simulink model "passive_cellBalancing"  (R2021a)
settings: Solver=VariableStepAuto  StartTime=0.0  StopTime=4000  RelTol=1e-3
undefined symbols (not defined in the file or in its folder): Ion, Lithium
libraries: spsBatteryLib x4, spsMosfetLib x4, spsSeriesRLCBranchLib x4, spspowerguiLib x1
settings Model: EnablePacing=on  PacingRate=100  Creator=Navadeep  LastModifiedBy=Navadeep

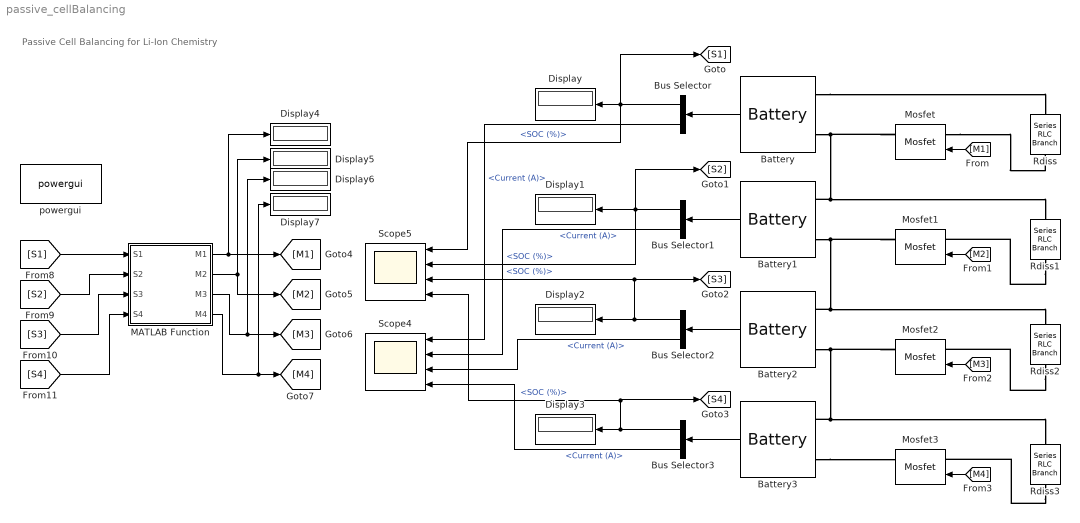
== system passive_cellBalancing ==
  note: Passive Cell Balancing for Li-Ion Chemistry
  Battery : spsBatteryLib/Battery  BatType=Lithium-Ion  ShowTempParam=off  ThermalPreset=no  ShowAgeParam=off  NomV=3.7  NomQ=7.5  SOC=70  Batt_Tr=30  PresetModel=on  MaxQ=7.5  MinV=2.775  FullV=4.3068  Dis_rate=3.2609  R=0.0049333  Normal_OP=6.7826  expZone="[3.9974     0.36848]"  current=[6.5 13 32.5]  Units=Time  Tci=20  NomT=20  T2=-30  MaxQ2=4.8  FullV2=7.1  Normal_OP2=5.655  expZone2="[6.58           1]"  Rca=0.6  ti=2000  Dp=0  Neq0=0  Tsim=1e6  Ta1=25  Qeol=5.4*0.9  Reol=0.013333*1.2  Char_age=[2.3478, 3]  Dis_age=[2.3478, 10]  N1=1500  N2=10500  N3=1000  N4=1400  Ta2=45  N5=950
  Battery1 : spsBatteryLib/Battery  BatType=Lithium-Ion  ShowTempParam=off  ThermalPreset=no  ShowAgeParam=off  NomV=3.7  NomQ=7.5  SOC=80  Batt_Tr=30  PresetModel=on  MaxQ=7.5  MinV=2.775  FullV=4.3068  Dis_rate=3.2609  R=0.0049333  Normal_OP=6.7826  expZone="[3.9974     0.36848]"  current=[6.5 13 32.5]  Units=Time  Tci=20  NomT=20  T2=-30  MaxQ2=4.8  FullV2=7.1  Normal_OP2=5.655  expZone2="[6.58           1]"  Rca=0.6  ti=2000  Dp=0  Neq0=0  Tsim=1e6  Ta1=25  Qeol=5.4*0.9  Reol=0.013333*1.2  Char_age=[2.3478, 3]  Dis_age=[2.3478, 10]  N1=1500  N2=10500  N3=1000  N4=1400  Ta2=45  N5=950
  Battery2 : spsBatteryLib/Battery  BatType=Lithium-Ion  ShowTempParam=off  ThermalPreset=no  ShowAgeParam=off  NomV=3.7  NomQ=7.5  SOC=75  Batt_Tr=30  PresetModel=on  MaxQ=7.5  MinV=2.775  FullV=4.3068  Dis_rate=3.2609  R=0.0049333  Normal_OP=6.7826  expZone="[3.9974     0.36848]"  current=[6.5 13 32.5]  Units=Time  Tci=20  NomT=20  T2=-30  MaxQ2=4.8  FullV2=7.1  Normal_OP2=5.655  expZone2="[6.58           1]"  Rca=0.6  ti=2000  Dp=0  Neq0=0  Tsim=1e6  Ta1=25  Qeol=5.4*0.9  Reol=0.013333*1.2  Char_age=[2.3478, 3]  Dis_age=[2.3478, 10]  N1=1500  N2=10500  N3=1000  N4=1400  Ta2=45  N5=950
  Battery3 : spsBatteryLib/Battery  BatType=Lithium-Ion  ShowTempParam=off  ThermalPreset=no  ShowAgeParam=off  NomV=3.7  NomQ=7.5  SOC=85  Batt_Tr=30  PresetModel=on  MaxQ=7.5  MinV=2.775  FullV=4.3068  Dis_rate=3.2609  R=0.0049333  Normal_OP=6.7826  expZone="[3.9974     0.36848]"  current=[6.5 13 32.5]  Units=Time  Tci=20  NomT=20  T2=-30  MaxQ2=4.8  FullV2=7.1  Normal_OP2=5.655  expZone2="[6.58           1]"  Rca=0.6  ti=2000  Dp=0  Neq0=0  Tsim=1e6  Ta1=25  Qeol=5.4*0.9  Reol=0.013333*1.2  Char_age=[2.3478, 3]  Dis_age=[2.3478, 10]  N1=1500  N2=10500  N3=1000  N4=1400  Ta2=45  N5=950
  Bus Selector{,1..3} (4 alike) : BusSelector  OutputSignals=SOC (%),Current (A)
  Display{,1..7} (8 alike) : Display
  MATLAB Function : MATLAB Function  TreatAsAtomicUnit=on
  Mosfet{,1..3} (4 alike) : spsMosfetLib/Mosfet  Ron=0.1  Lon=0  Rd=0.01  Vfd=0  IC=0  Rs=1e5  Cs=inf  Measurements=on
  Rdiss : spsSeriesRLCBranchLib/Series RLC Branch  LConnTagsString=__new0  RConnTagsString=__new0  BranchType=R  Resistance=1  Inductance=1e-3  SetiL0=off  InitialCurrent=0  Capacitance=1e-6  Setx0=off  InitialVoltage=0  Measurements=None
  Rdiss1 : spsSeriesRLCBranchLib/Series RLC Branch  LConnTagsString=__new0  RConnTagsString=__new0  BranchType=R  Resistance=4  Inductance=1e-3  SetiL0=off  InitialCurrent=0  Capacitance=1e-6  Setx0=off  InitialVoltage=0  Measurements=None
  Rdiss2 : spsSeriesRLCBranchLib/Series RLC Branch  LConnTagsString=__new0  RConnTagsString=__new0  BranchType=R  Resistance=5  Inductance=1e-3  SetiL0=off  InitialCurrent=0  Capacitance=1e-6  Setx0=off  InitialVoltage=0  Measurements=None
  Rdiss3 : spsSeriesRLCBranchLib/Series RLC Branch  LConnTagsString=__new0  RConnTagsString=__new0  BranchType=R  Resistance=5  Inductance=1e-3  SetiL0=off  InitialCurrent=0  Capacitance=1e-6  Setx0=off  InitialVoltage=0  Measurements=None
  Scope4 : Scope  NumInputPorts=4
  Scope5 : Scope  NumInputPorts=4
  powergui : spspowerguiLib/powergui  Priority=1  SimulationMode=Discrete  SampleTime=0.05  frequency=60  Iterations=50  frequencyindice=0  Pbase=100e6  ErrMax=1e-4  UnitsV=kV  UnitsW=MW  buscounter=0  FunctionMessages=off  echomessages=off  EnableUseOfTLC=off  CurrentSourceSwitches=off  DisableSnubberDevices=off  DisableRonSwitches=off  DisableVfSwitches=off  DisplayEquations=off  AutomaticDiscreteSolvers=off  SolverType=Tustin/Backward Euler (TBE)  Interpol=off  ExternalGateDelay=off  methode=off  Ts=100  x0status=blocks  SPID=on  SwTol=0  HookPort=off  NonlinearTolerance=1e-4  nMaxIteration=100  ContinueOnMaxIteration=off  RestoreLinks=warning  ResistiveCurrentMeasurement=off  Frange=[0:2:500]  Ylog=off  Xlog=on  ShowGrid=off  save=off  variable=ZData  structure=0  ZoomFFT=off  StartTime=0.0  cycles=1  DisplayStyle=1  fundamental=60  FreqAxis=off  MaxFrequency=1000  frequencyindicesteady=1  RmsSteady=1  display=off
  wires:
  Battery/1 -> Bus Selector/1
  Bus Selector/1 -> [S1], Display/1, Scope5/1  "<SOC (%)>"
  Battery1/1 -> Bus Selector1/1
  Bus Selector1/1 -> Display1/1, [S2], Scope5/2  "<SOC (%)>"
  Battery2/1 -> Bus Selector2/1
  Bus Selector2/1 -> Display2/1, [S3], Scope5/3  "<SOC (%)>"
  Battery3/1 -> Bus Selector3/1
  Bus Selector3/1 -> Display3/1, [S4], Scope5/4  "<SOC (%)>"
  Bus Selector/2 -> Scope4/1  "<Current (A)>"
  Bus Selector1/2 -> Scope4/2  "<Current (A)>"
  Bus Selector2/2 -> Scope4/3  "<Current (A)>"
  Bus Selector3/2 -> Scope4/4  "<Current (A)>"
  [M2] -> Mosfet1/1
  [M1] -> Mosfet/1
  [M3] -> Mosfet2/1
  [M4] -> Mosfet3/1
  [S1] -> MATLAB Function/1(S1)
  [S2] -> MATLAB Function/2(S2)
  [S3] -> MATLAB Function/3(S3)
  [S4] -> MATLAB Function/4(S4)
  MATLAB Function/1(M1) -> [M1], Display4/1
  MATLAB Function/2(M2) -> [M2], Display5/1
  MATLAB Function/3(M3) -> Display6/1, [M3]
  MATLAB Function/4(M4) -> Display7/1, [M4]
  connections:
  Battery/LConn2 -- Rdiss1/RConn1 -- Battery1/LConn1 -- Mosfet/RConn1
  Battery1/LConn2 -- Rdiss2/RConn1 -- Battery2/LConn1 -- Mosfet1/RConn1
  Battery2/LConn2 -- Mosfet2/RConn1 -- Rdiss3/RConn1 -- Battery3/LConn1
  Battery3/LConn2 -- Mosfet3/RConn1
  Battery/LConn1 -- Rdiss/RConn1
  Rdiss1/LConn1 -- Mosfet1/LConn1
  Rdiss2/LConn1 -- Mosfet2/LConn1
  Rdiss3/LConn1 -- Mosfet3/LConn1
  Mosfet/LConn1 -- Rdiss/LConn1

== matlab function passive_cellBalancing/MATLAB Function ==
  data: S1 input; M1 output; S2 input; S3 input; M2 output; M3 output; S4 input; M4 output
%function to control the triggering of MOSFETs M1:M4
function [M1, M2, M3, M4] = fcn(S1, S2, S3, S4)

%input the SOC values from individual cells
S1 = int16(S1);
S2 = int16(S2);
S3 = int16(S3);
S4 = int16(S4);

%initial definitions for MOSFET states
M1 = 0;
M2 = 0;
M3 = 0;
M4 = 0;

%find the minimum SOC 
minSOC= min([S1 S2 S3 S4]);

%check if there is a SOC imbalance
if(~isequal(S1, S2 ,S3, S4))
    
%case1
if(S1 == minSOC)
    if(S2==minSOC)
        if(S3==minSOC)
            M4 = 1;
        elseif(S4==minSOC)
            M3 = 1;
        else 
            M3 = 1;
            M4 = 1;
        end
        
    elseif(S3==minSOC)
        if(S4==minSOC)
            M2 = 1;
        elseif(S1==minSOC)
            M2 = 1;
            M4 = 1;
        end
        
    elseif(S4==minSOC)
            M2 = 1;
            M3 = 1;
    else
            M2 = 1;
            M3 = 1;
            M4 = 1;
    end

%case2
elseif(S2 == minSOC)
    if(S3==minSOC)
        if(S1==minSOC)
            M4 = 1;
        elseif(S4==minSOC)
            M1 = 1;
        else
            M1 = 1;
            M4 = 1;
        end
        
    elseif(S4==minSOC)
        if(S1==minSOC)
            M3 = 1;
        elseif(S2==minSOC)
            M1 = 1;
            M3 = 1;
        end
        
    elseif(S1==minSOC)
        M3 = 1;
        M4 = 1;
        
    else
        M1 = 1;
        M3 = 1;
        M4 = 1;
    end

%case3
elseif(S3 == minSOC)
    if(S1==minSOC)
        if(S2==minSOC)
            M4 = 1;
        elseif(S4==minSOC)
            M2 = 1;
        else
            M2 = 1;
            M4 = 1;
        end
        
    elseif(S4==minSOC)
        if(S2==minSOC)
            M1 = 1;
        else
            M1 = 1;
            M2 = 1;
        end
    elseif(S2==minSOC)
        M1 = 1;
        M4 = 1;
        
    else
        M1 = 1;
        M2 = 1;
        M4 = 1;
    end

%case4
elseif(S4 == minSOC)
    if(S1==minSOC)
        if(S2==minSOC)
            M3 = 1;
       
        elseif(S3==minSOC)
            M2 = 1;
            
        else
            M2 = 1;
            M3 = 1;
        end
        
     elseif(S2==minSOC)
         if(S3==minSOC)
            M1 = 1;
            
         else
            M1 = 1;
            M2 = 1;
         end
         
    elseif(S3 == minSOC)
        M1 = 1;
        M2 = 1;
        
    else
        M1 = 1;
        M2 = 1;
        M3 = 1;
    end
end
end
end
